simulink model "model_airfoil_version2"  (R2024b)
settings: Solver=VariableStepAuto  StartTime=0.0  StopTime=4  RelTol=1e-3
model workspace (MAT data in the model file):
  k1 = 0
  k2 = 0
  k_d = 0
  k_p = 0
values from neighbouring files (symbols this model uses):
  c_d = 200    [init_params.m]
  I = 1e2    (= 100)    [init_params.m]
libraries: simulink x2
settings Model: Creator=Randy  LastModifiedBy=Randy
settings DebuggingCC: AlgebraicLoopMsg=none

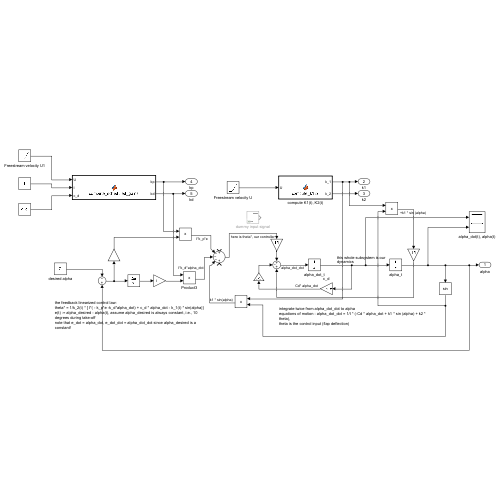
[thumbnail: Simulink's stored preview of the top-level diagram]
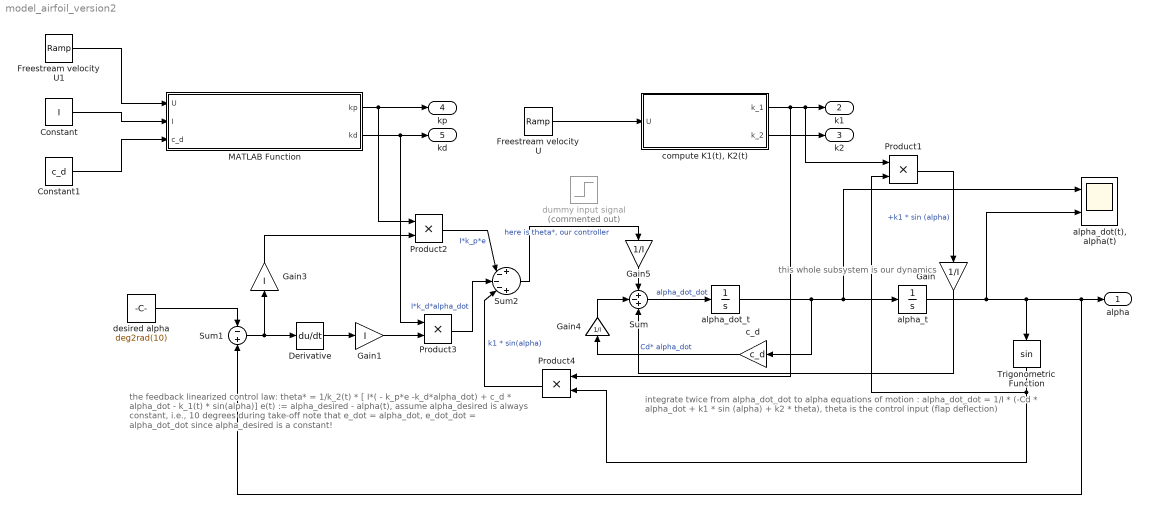
== system model_airfoil_version2 ==
  note: this whole subsystem is our dynamics
  note: the feedback linearized control law:
      | theta* = 1/k_2(t) * [ I*( - k_p*e -k_d*alpha_dot) + c_d * alpha_dot - k_1(t) * sin(alpha)]
      | e(t) := alpha_desired - alpha(t), assume alpha_desired is always constant, i.e., 10 degrees during take-off
      | note that e_dot = alpha_dot, e_dot_dot = alpha_dot_dot since alpha_desired is a constant!
  note: integrate twice from alpha_dot_dot to alpha
      | equations of motion : alpha_dot_dot = 1/I * (-Cd * alpha_dot + k1 * sin (alpha) + k2 * theta),
      | theta is the control input (flap deflection)
  Constant : Constant  Value=I
  Constant1 : Constant  Value=c_d
  Derivative : Derivative
  Freestream velocity U : simulink/Sources/Ramp  slope=5  start=0.5  InitialOutput=15
  Freestream velocity U1 : simulink/Sources/Ramp  slope=5  start=0.5  InitialOutput=15
  Gain : Gain  Gain=1/I
  Gain1 : Gain  Gain=I
  Gain3 : Gain  Gain=I
  Gain4 : Gain  Gain=1/I
  Gain5 : Gain  Gain=1/I
  MATLAB Function : MATLAB Function  TreatAsAtomicUnit=on
  Product{1..4} (4 alike) : Product
  Sum : Sum  Inputs=+-+
  Sum1 : Sum  Inputs=-+
  Sum2 : Sum  Inputs=+---+
  Trigonometric Function : Trigonometry
  "alpha_dot(t), alpha(t)" : Scope  NumInputPorts=2
  alpha_dot_t : Integrator
  alpha_t : Integrator
  c_d : Gain  Gain=c_d
  "compute K1(t), K2(t)" : MATLAB Function  TreatAsAtomicUnit=on
  desired alpha : Constant  Value=deg2rad(10)
  dummy input signal : Step  Commented=on  SampleTime=0
  alpha : Outport
  k1 : Outport  Port=2
  k2 : Outport  Port=3
  kp : Outport  Port=4
  kd : Outport  Port=5
  wires:
  Freestream velocity U/1 -> "compute K1(t), K2(t)"/1(U)
  alpha_dot_t/1 -> alpha_t/1, "alpha_dot(t), alpha(t)"/1, c_d/1
  alpha_t/1 -> Sum1/2, alpha/1, Trigonometric Function/1, "alpha_dot(t), alpha(t)"/2
  "compute K1(t), K2(t)"/1(k_1) -> k1/1, Product1/1, Product4/1
  "compute K1(t), K2(t)"/2(k_2) -> k2/1
  Sum/1 -> alpha_dot_t/1  "alpha_dot_dot"
  desired alpha/1 -> Sum1/1
  Constant/1 -> MATLAB Function/2(I)
  Constant1/1 -> MATLAB Function/3(c_d)
  Freestream velocity U1/1 -> MATLAB Function/1(U)
  MATLAB Function/1(kp) -> Product2/1, kp/1
  MATLAB Function/2(kd) -> Product3/1, kd/1
  Sum1/1 -> Derivative/1, Gain3/1
  Gain3/1 -> Product2/2
  Product2/1 -> Sum2/2  "I*k_p*e"
  Product3/1 -> Sum2/3  "I*k_d*alpha_dot"
  Trigonometric Function/1 -> Product1/2, Product4/2
  Gain1/1 -> Product3/2
  Product4/1 -> Sum2/4  "k1 * sin(alpha)"
  c_d/1 -> Gain4/1  "Cd* alpha_dot"
  Gain4/1 -> Sum/2
  Product1/1 -> Gain/1  "+k1 * sin (alpha)"
  Gain/1 -> Sum/3
  Gain5/1 -> Sum/1
  Sum2/1 -> Gain5/1  "here is theta*, our controller"
  Derivative/1 -> Gain1/1

== matlab function model_airfoil_version2/MATLAB Function ==
  data: U input; kp output; I input; c_d input; kd output
function [kp, kd] = compute_scheduled_gains(U, I, c_d)
    % Schedule omega_n based on U(t) (e.g., higher speed → faster response)
    %omega_n = 1 + 0.1 * U;  % Example: Increase omega_n with U(t)
    omega_n = 2.0;
    zeta = 0.9;              % Fixed damping ratio-> minimum overshoot
    
    kp = omega_n^2 * I;
    kd = 2 * zeta * omega_n * I;
end

== matlab function model_airfoil_version2/compute K1(t), K2(t) ==
  data: U input; k_1 output; k_2 output
function [k_1, k_2] = compute_k1k2(U)
    rho = 1.225;    % Air density (kg/m³)
    S = 5;         % Wing area (m²)
    c = 2;          % Chord length (m)
    d = 0.5;        % Pivot-to-AC distance (m)
    Cmd = -0.1;     % Flap effectiveness coefficient
    
    k_1 = pi * rho * U^2 * S * d;
    k_2 = 0.5 * rho * U^2 * S * c * Cmd;
end
